simulink model "Mohinhmoix"  (R2018a)
settings: Solver=ode5  StartTime=0.0  StopTime=100  FixedStep=0.05  RelTol=1e-3
libraries: simulink x2
settings Model: PacingRate=10  Creator=Hungs  LastModifiedBy=Hungs

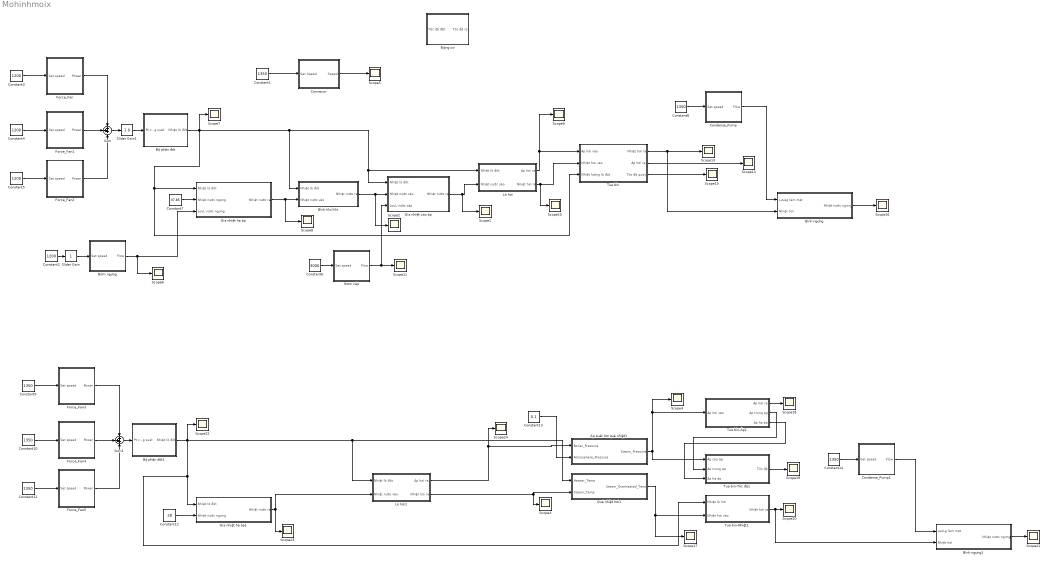
== system Mohinhmoix ==
  Bình khử khí : Subsystem
  Bình ngưng : Subsystem
  Bình ngưng1 : Subsystem
  Bơm cấp : Subsystem
      mask Display: image('C:\Program Files\MATLAB\ThermalElectricity\Maskicon\Pump.png');
  Bơm ngưng : Subsystem
      mask Display: image('C:\Program Files\MATLAB\ThermalElectricity\Maskicon\Pump.png');
  Bộ phận đốt : Subsystem
      mask Display: image('C:\Program Files\MATLAB\ThermalElectricity\Maskicon\Furnace.png');
  Bộ phận đốt1 : Subsystem
      mask Display: image('C:\Program Files\MATLAB\ThermalElectricity\Maskicon\Furnace.png');
  Condense_Pump : Subsystem
      mask Display: image('C:\Program Files\MATLAB\ThermalElectricity\Maskicon\Pump.png');
  Condense_Pump1 : Subsystem
      mask Display: image('C:\Program Files\MATLAB\ThermalElectricity\Maskicon\Pump.png');
  Constant{1,8..11,14} (6 alike) : Constant  Value=1350
  Constant12 : Constant  Value=28
  Constant13 : Constant  Value=0.1
  Constant{2..5} (4 alike) : Constant  Value=1200
  Constant6 : Constant  Value=3000
  Constant7 : Constant  Value=37.85
  Conveyor : Subsystem
      mask Display: image('C:\Program Files\MATLAB\ThermalElectricity\Maskicon\conveyor.png');
  Force_Fan : Subsystem
      mask Display: image('C:\Program Files\MATLAB\ThermalElectricity\Maskicon\Fan.png');
  Force_Fan1 : Subsystem
      mask Display: image('C:\Program Files\MATLAB\ThermalElectricity\Maskicon\Fan.png');
  Force_Fan2 : Subsystem
      mask Display: image('C:\Program Files\MATLAB\ThermalElectricity\Maskicon\Fan.png');
  Force_Fan3 : Subsystem
      mask Display: image('C:\Program Files\MATLAB\ThermalElectricity\Maskicon\Fan.png');
  Force_Fan4 : Subsystem
      mask Display: image('C:\Program Files\MATLAB\ThermalElectricity\Maskicon\Fan.png');
  Force_Fan5 : Subsystem
      mask Display: image('C:\Program Files\MATLAB\ThermalElectricity\Maskicon\Fan.png');
  Gia nhiệt cao áp : Subsystem
  Gia nhiệt hạ áp : Subsystem
  Gia nhiệt hạ áp1 : Subsystem
  Lò hơi : Subsystem
  Lò hơi1 : Subsystem
  Quá nhiệt hơi1 : Subsystem
  Scope{1..11,13..24} (23 alike) : Scope
  Slider Gain : simulink/Math Operations/Slider Gain  gain=1  low=0  high=2
  Slider Gain1 : simulink/Math Operations/Slider Gain  gain=1.0  low=0  high=2
  Sum : Sum  Inputs=+++
  Sum1 : Sum  Inputs=+++
  Tua bin : Subsystem
  Tua bin-Nhiệt1 : Subsystem
  Tua bin-Tốc độ1 : Subsystem
  Tua bin-Áp1 : Subsystem
  Áp suất hơi quá nhiệt1 : Subsystem
  Động cơ : Subsystem
  wires:
  Constant1/1 -> Conveyor/1(Set Speed)
  Conveyor/1(Speed) -> Scope5/1
  Constant2/1 -> Slider Gain/1
  Bơm ngưng/1(Flow) -> Scope6/1, Gia nhiệt hạ áp/3(LưuL nước ngưng)
  Force_Fan/1(Power) -> Sum/1
  Constant3/1 -> Force_Fan/1(Set speed)
  Constant4/1 -> Force_Fan1/1(Set speed)
  Force_Fan2/1(Power) -> Sum/3
  Constant5/1 -> Force_Fan2/1(Set speed)
  Sum/1 -> Slider Gain1/1
  Force_Fan1/1(Power) -> Sum/2
  Lò hơi/1(Áp hơi ra) -> Scope9/1, Tua bin/1(Áp hơi vào)
  Lò hơi/2(Nhiệt hơi ra) -> Scope10/1, Tua bin/2(Nhiệt hơi vào)
  Tua bin/1(Nhiệt hơi ra) -> Bình ngưng/2(Nhiệt hơi), Scope13/1
  Tua bin/2(Áp hơi ra) -> Scope14/1
  Tua bin/3(Tốc độ quay) -> Scope15/1
  Constant8/1 -> Condense_Pump/1(Set speed)
  Condense_Pump/1(Flow) -> Bình ngưng/1(LưuLg làm mát)
  Bình ngưng/1(Nhiệt nước ngưng) -> Scope16/1
  Constant12/1 -> Gia nhiệt hạ áp1/2(Nhiệt nước ngưng)
  Bình ngưng1/1(Nhiệt nước ngưng) -> Scope21/1
  Constant14/1 -> Condense_Pump1/1(Set speed)
  Tua bin-Nhiệt1/1(Nhiệt hơi ra) -> Bình ngưng1/2(Nhiệt hơi), Scope20/1
  Lò hơi1/2(Nhiệt hơi ra) -> Quá nhiệt hơi1/2(Steam_Temp), Scope3/1
  Constant10/1 -> Force_Fan4/1(Set speed)
  Tua bin-Áp1/1(Áp hơi ra) -> Scope18/1
  Constant11/1 -> Force_Fan5/1(Set speed)
  Condense_Pump1/1(Flow) -> Bình ngưng1/1(LưuLg làm mát)
  Force_Fan5/1(Power) -> Sum1/3
  Bộ phận đốt1/1(Nhiệt lò đốt) -> Quá nhiệt hơi1/1(Heater_Temp), Lò hơi1/1(Nhiệt lò đốt), Tua bin-Nhiệt1/1(Nhiệt lò hơi), Gia nhiệt hạ áp1/1(Nhiệt lò đốt), Scope22/1
  Quá nhiệt hơi1/1(Steam_Overheated_Temp) -> Tua bin-Nhiệt1/2(Nhiệt hơi vào), Scope17/1
  Constant13/1 -> Áp suất hơi quá nhiệt1/2(Atmosphere_Pressure)
  Tua bin-Áp1/3(Áp hạ áp) -> Tua bin-Tốc độ1/3(Áp hạ áp)
  Force_Fan4/1(Power) -> Sum1/2
  Áp suất hơi quá nhiệt1/1(Steam_Pressure) -> Tua bin-Tốc độ1/1(Áp cao áp), Tua bin-Áp1/1(Áp hơi vào), Scope4/1
  Gia nhiệt hạ áp1/1(Nhiệt nước ra) -> Lò hơi1/2(Nhiệt nước vào), Scope23/1
  Constant9/1 -> Force_Fan3/1(Set speed)
  Sum1/1 -> Bộ phận đốt1/1(Pt công suất)
  Force_Fan3/1(Power) -> Sum1/1
  Lò hơi1/1(Áp hơi ra) -> Áp suất hơi quá nhiệt1/1(Boiler_Pressure), Scope24/1
  Tua bin-Áp1/2(Áp trung áp) -> Tua bin-Tốc độ1/2(Áp trung áp)
  Tua bin-Tốc độ1/1(Tốc độ) -> Scope19/1
  Constant7/1 -> Gia nhiệt hạ áp/2(Nhiệt nước ngưng)
  Slider Gain/1 -> Bơm ngưng/1(Set speed)
  Slider Gain1/1 -> Bộ phận đốt/1(Pt công suất)
  Bộ phận đốt/1(Nhiệt lò đốt) -> Bình khử khí/1(Nhiệt lò đốt), Lò hơi/1(Nhiệt lò đốt), Gia nhiệt cao áp/1(Nhiệt lò đốt), Tua bin/3(Nhiệt lượng lò đốt), Gia nhiệt hạ áp/1(Nhiệt lò đốt), Scope7/1
  Gia nhiệt hạ áp/1(Nhiệt nước ra) -> Bình khử khí/2(Nhiệt nước vào), Scope8/1
  Bình khử khí/1(Nhiệt nước ra) -> Scope2/1, Gia nhiệt cao áp/2(Nhiệt nước vào)
  Constant6/1 -> Bơm cấp/1(Set speed)
  Bơm cấp/1(Flow) -> Scope11/1, Gia nhiệt cao áp/3(LưuL nước cấp)
  Gia nhiệt cao áp/1(Nhiệt nước ra) -> Scope1/1, Lò hơi/2(Nhiệt nước vào)

== system Mohinhmoix/Bình khử khí ==
  Nhiệt lò đốt : Inport
  Nhiệt nước vào : Inport  Port=2
  Gia nhiệt cao áp : TransferFcn  Numerator=[0.0435]  Denominator=[8 1]
  Sum : Sum  Inputs=|++
  Nhiệt nước ra : Outport
  wires:
  Nhiệt lò đốt/1 -> Gia nhiệt cao áp/1
  Nhiệt nước vào/1 -> Sum/1
  Gia nhiệt cao áp/1 -> Sum/2
  Sum/1 -> Nhiệt nước ra/1

== system Mohinhmoix/Bình ngưng ==
  LưuLg làm mát : Inport
  Nhiệt hơi : Inport  Port=2
  Ngưng tụ : TransferFcn  Numerator=[4.454]  Denominator=[12 1]
  Sum : Sum  Inputs=|+-
  Nhiệt nước ngưng : Outport
  wires:
  Sum/1 -> Nhiệt nước ngưng/1
  Ngưng tụ/1 -> Sum/2
  Nhiệt hơi/1 -> Sum/1
  LưuLg làm mát/1 -> Ngưng tụ/1

== system Mohinhmoix/Bình ngưng1 ==
  LưuLg làm mát : Inport
  Nhiệt hơi : Inport  Port=2
  Ngưng tụ : TransferFcn  Numerator=[5]  Denominator=[12 1]
  Sum : Sum  Inputs=|+-
  Nhiệt nước ngưng : Outport
  wires:
  Sum/1 -> Nhiệt nước ngưng/1
  Ngưng tụ/1 -> Sum/2
  Nhiệt hơi/1 -> Sum/1
  LưuLg làm mát/1 -> Ngưng tụ/1

== system Mohinhmoix/Bơm cấp ==
  Set speed : Inport
  Heat_Flow : TransferFcn  Numerator=[0.195]  Denominator=[10 1]
  Motor : TransferFcn  Denominator=[1 1 1]
  Flow : Outport
  wires:
  Motor/1 -> Heat_Flow/1
  Set speed/1 -> Motor/1
  Heat_Flow/1 -> Flow/1

== system Mohinhmoix/Bơm ngưng ==
  Set speed : Inport
  Heat_Flow : TransferFcn  Numerator=[0.512]  Denominator=[10 1]
  Motor : TransferFcn  Denominator=[1 1 1]
  Flow : Outport
  wires:
  Heat_Flow/1 -> Flow/1
  Set speed/1 -> Motor/1
  Motor/1 -> Heat_Flow/1

== system Mohinhmoix/Bộ phận đốt ==
  Pt công suất : Inport
  Vòi đốt : TransferFcn  Numerator=[1687.5]  Denominator=[5 1]
  Nhiệt lò đốt : Outport
  wires:
  Vòi đốt/1 -> Nhiệt lò đốt/1
  Pt công suất/1 -> Vòi đốt/1

== system Mohinhmoix/Bộ phận đốt1 ==
  Pt công suất : Inport
  Vòi đốt : TransferFcn  Numerator=[1350]  Denominator=[5 1]
  Nhiệt lò đốt : Outport
  wires:
  Vòi đốt/1 -> Nhiệt lò đốt/1
  Pt công suất/1 -> Vòi đốt/1

== system Mohinhmoix/Condense_Pump ==
  Set speed : Inport
  Condense_Flow : TransferFcn  Numerator=[0.012]  Denominator=[6 1]
  Motor : TransferFcn  Denominator=[1 1 1]
  Flow : Outport
  wires:
  Motor/1 -> Condense_Flow/1
  Set speed/1 -> Motor/1
  Condense_Flow/1 -> Flow/1

== system Mohinhmoix/Condense_Pump1 ==
  Set speed : Inport
  Condense_Flow : TransferFcn  Numerator=[0.012]  Denominator=[6 1]
  Motor : TransferFcn  Denominator=[1 1 1]
  Flow : Outport
  wires:
  Motor/1 -> Condense_Flow/1
  Set speed/1 -> Motor/1
  Condense_Flow/1 -> Flow/1

== system Mohinhmoix/Conveyor ==
  Set Speed : Inport
  Motor_1 : TransferFcn  Denominator=[1 1 1]
  Speed : Outport
  wires:
  Set Speed/1 -> Motor_1/1
  Motor_1/1 -> Speed/1

== system Mohinhmoix/Force_Fan ==
  Set speed : Inport
  Heat_Power : TransferFcn  Numerator=[0.000222]  Denominator=[3 1]
  Motor : TransferFcn  Denominator=[1 1 1]
  Power : Outport
  wires:
  Motor/1 -> Heat_Power/1
  Set speed/1 -> Motor/1
  Heat_Power/1 -> Power/1

== system Mohinhmoix/Force_Fan1 ==
  Set speed : Inport
  Heat_Power : TransferFcn  Numerator=[0.000222]  Denominator=[3 1]
  Motor : TransferFcn  Denominator=[1 1 1]
  Power : Outport
  wires:
  Heat_Power/1 -> Power/1
  Set speed/1 -> Motor/1
  Motor/1 -> Heat_Power/1

== system Mohinhmoix/Force_Fan2 ==
  Set speed : Inport
  Heat_Power : TransferFcn  Numerator=[0.000222]  Denominator=[3 1]
  Motor : TransferFcn  Denominator=[1 1 1]
  Power : Outport
  wires:
  Motor/1 -> Heat_Power/1
  Set speed/1 -> Motor/1
  Heat_Power/1 -> Power/1

== system Mohinhmoix/Force_Fan3 ==
  Set speed : Inport
  Heat_Power : TransferFcn  Numerator=[0.00025]  Denominator=[3 1]
  Motor : TransferFcn  Denominator=[1 1 1]
  Power : Outport
  wires:
  Motor/1 -> Heat_Power/1
  Set speed/1 -> Motor/1
  Heat_Power/1 -> Power/1

== system Mohinhmoix/Force_Fan4 ==
  Set speed : Inport
  Heat_Power : TransferFcn  Numerator=[0.00025]  Denominator=[3 1]
  Motor : TransferFcn  Denominator=[1 1 1]
  Power : Outport
  wires:
  Heat_Power/1 -> Power/1
  Set speed/1 -> Motor/1
  Motor/1 -> Heat_Power/1

== system Mohinhmoix/Force_Fan5 ==
  Set speed : Inport
  Heat_Power : TransferFcn  Numerator=[0.00025]  Denominator=[3 1]
  Motor : TransferFcn  Denominator=[1 1 1]
  Power : Outport
  wires:
  Motor/1 -> Heat_Power/1
  Set speed/1 -> Motor/1
  Heat_Power/1 -> Power/1

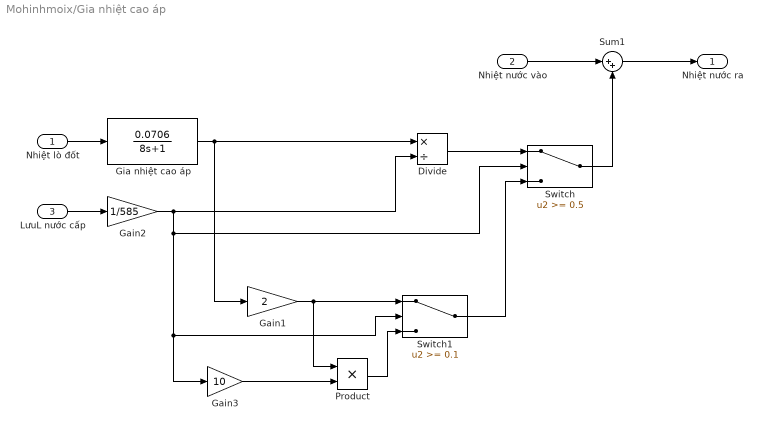
== system Mohinhmoix/Gia nhiệt cao áp ==
  Nhiệt lò đốt : Inport
  Nhiệt nước vào : Inport  Port=2
  LưuL nước cấp : Inport  Port=3
  Divide : Product  Inputs=*/
  Gain1 : Gain  Gain=2
  Gain2 : Gain  Gain=1/585
  Gain3 : Gain  Gain=10
  Gia nhiệt cao áp : TransferFcn  Numerator=[0.0706]  Denominator=[8 1]
  Product : Product
  Sum1 : Sum  Inputs=|++
  Switch : Switch  Threshold=0.5
  Switch1 : Switch  Threshold=0.1
  Nhiệt nước ra : Outport
  wires:
  Nhiệt lò đốt/1 -> Gia nhiệt cao áp/1
  Switch1/1 -> Switch/3
  Sum1/1 -> Nhiệt nước ra/1
  Switch/1 -> Sum1/2
  Nhiệt nước vào/1 -> Sum1/1
  Gain1/1 -> Switch1/1, Product/1
  Gain3/1 -> Product/2
  Product/1 -> Switch1/3
  Gia nhiệt cao áp/1 -> Divide/1, Gain1/1
  Gain2/1 -> Gain3/1, Switch1/2, Switch/2, Divide/2
  LưuL nước cấp/1 -> Gain2/1
  Divide/1 -> Switch/1

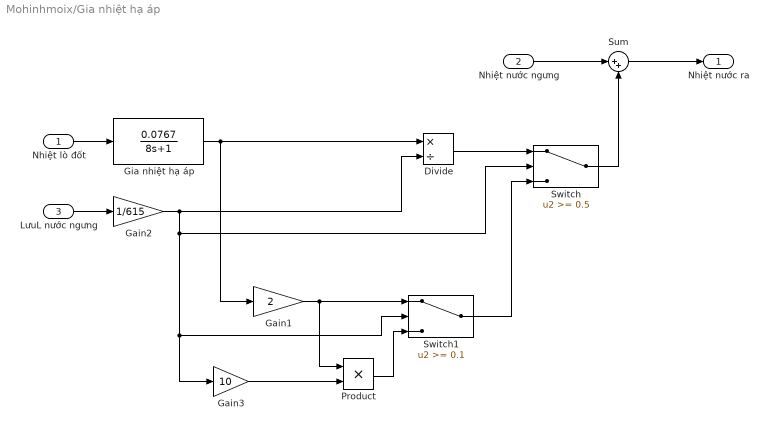
== system Mohinhmoix/Gia nhiệt hạ áp ==
  Nhiệt lò đốt : Inport
  Nhiệt nước ngưng : Inport  Port=2
  LưuL nước ngưng : Inport  Port=3
  Divide : Product  Inputs=*/
  Gain1 : Gain  Gain=2
  Gain2 : Gain  Gain=1/615
  Gain3 : Gain  Gain=10
  Gia nhiệt hạ áp : TransferFcn  Numerator=[0.0767]  Denominator=[8 1]
  Product : Product
  Sum : Sum  Inputs=|++
  Switch : Switch  Threshold=0.5
  Switch1 : Switch  Threshold=0.1
  Nhiệt nước ra : Outport
  wires:
  Sum/1 -> Nhiệt nước ra/1
  Nhiệt nước ngưng/1 -> Sum/1
  Nhiệt lò đốt/1 -> Gia nhiệt hạ áp/1
  Gia nhiệt hạ áp/1 -> Divide/1, Gain1/1
  Gain2/1 -> Gain3/1, Switch1/2, Switch/2, Divide/2
  Gain1/1 -> Switch1/1, Product/1
  Switch1/1 -> Switch/3
  Gain3/1 -> Product/2
  Product/1 -> Switch1/3
  Divide/1 -> Switch/1
  Switch/1 -> Sum/2
  LưuL nước ngưng/1 -> Gain2/1

== system Mohinhmoix/Gia nhiệt hạ áp1 ==
  Nhiệt lò đốt : Inport
  Nhiệt nước ngưng : Inport  Port=2
  Gia nhiệt hạ áp : TransferFcn  Numerator=[0.053]  Denominator=[8 1]
  Sum : Sum  Inputs=|++
  Nhiệt nước ra : Outport
  wires:
  Nhiệt lò đốt/1 -> Gia nhiệt hạ áp/1
  Nhiệt nước ngưng/1 -> Sum/1
  Gia nhiệt hạ áp/1 -> Sum/2
  Sum/1 -> Nhiệt nước ra/1

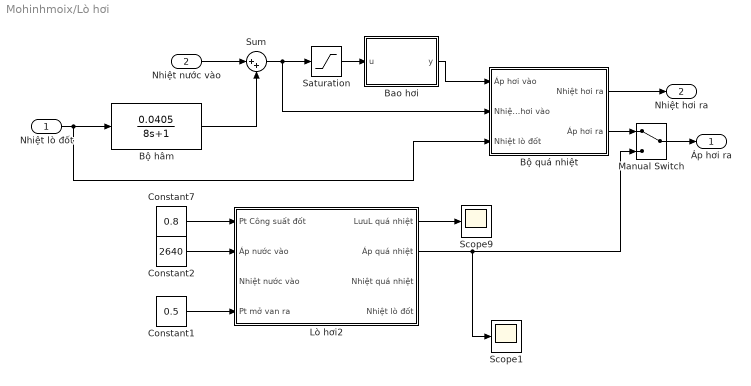
== system Mohinhmoix/Lò hơi ==
  Nhiệt lò đốt : Inport
  Nhiệt nước vào : Inport  Port=2
  Bao hơi : MATLAB Function  TreatAsAtomicUnit=on
  Bộ hâm : TransferFcn  Numerator=[0.0405]  Denominator=[8 1]
  Bộ quá nhiệt : Subsystem
  Constant1 : Constant  Value=0.5
  Constant2 : Constant  Value=2640
  Constant7 : Constant  Value=0.8
  Lò hơi2 : Subsystem
  Manual Switch : ManualSwitch
  Saturation : Saturate  UpperLimit=425  LowerLimit=0
  Scope1 : Scope
  Scope9 : Scope
  Sum : Sum  Inputs=|++
  Áp hơi ra : Outport
  Nhiệt hơi ra : Outport  Port=2
  wires:
  Sum/1 -> Bộ quá nhiệt/2(Nhiệt hơi vào), Saturation/1
  Bộ hâm/1 -> Sum/2
  Nhiệt nước vào/1 -> Sum/1
  Nhiệt lò đốt/1 -> Bộ quá nhiệt/3(Nhiệt lò đốt), Bộ hâm/1
  Bao hơi/1(y) -> Bộ quá nhiệt/1(Áp hơi vào)
  Bộ quá nhiệt/1(Nhiệt hơi ra) -> Nhiệt hơi ra/1
  Saturation/1 -> Bao hơi/1(u)
  Constant7/1 -> Lò hơi2/1(Pt Công suất đốt)
  Constant1/1 -> Lò hơi2/4(Pt mở van ra)
  Constant2/1 -> Lò hơi2/2(Áp nước vào)
  Lò hơi2/2(Áp quá nhiệt) -> Manual Switch/2, Scope1/1
  Lò hơi2/1(LưuL quá nhiệt) -> Scope9/1
  Bộ quá nhiệt/2(Áp hơi ra) -> Manual Switch/1
  Manual Switch/1 -> Áp hơi ra/1

== system Mohinhmoix/Lò hơi1 ==
  Nhiệt lò đốt : Inport
  Nhiệt nước vào : Inport  Port=2
  Bao hơi : MATLAB Function  TreatAsAtomicUnit=on
  Bộ hâm : TransferFcn  Numerator=[0.185]  Denominator=[8 1]
  Sum : Sum  Inputs=|++
  Áp hơi ra : Outport
  Nhiệt hơi ra : Outport  Port=2
  wires:
  Sum/1 -> Nhiệt hơi ra/1, Bao hơi/1(u)
  Bộ hâm/1 -> Sum/2
  Nhiệt nước vào/1 -> Sum/1
  Nhiệt lò đốt/1 -> Bộ hâm/1
  Bao hơi/1(y) -> Áp hơi ra/1

== system Mohinhmoix/Quá nhiệt hơi1 ==
  Heater_Temp : Inport
  Steam_Temp : Inport  Port=2
  Sum : Sum  Inputs=|++
  Water_Heat_Absorbing : TransferFcn  Numerator=[0.146]  Denominator=[6 1]
  Steam_Overheated_Temp : Outport
  wires:
  Sum/1 -> Steam_Overheated_Temp/1
  Water_Heat_Absorbing/1 -> Sum/2
  Steam_Temp/1 -> Sum/1
  Heater_Temp/1 -> Water_Heat_Absorbing/1

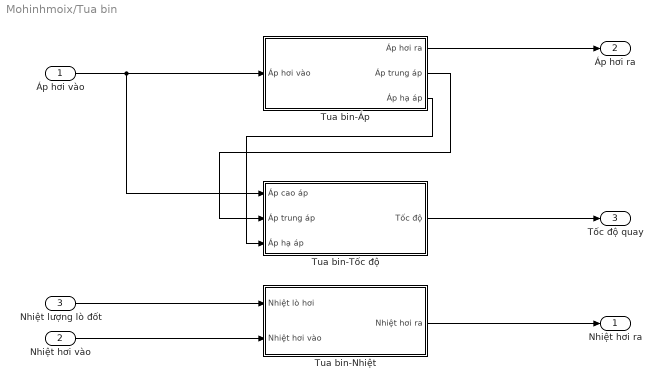
== system Mohinhmoix/Tua bin ==
  Áp hơi vào : Inport
  Nhiệt hơi vào : Inport  Port=2
  Nhiệt lượng lò đốt : Inport  Port=3
  Tua bin-Nhiệt : Subsystem
  Tua bin-Tốc độ : Subsystem
  Tua bin-Áp : Subsystem
  Nhiệt hơi ra : Outport
  Áp hơi ra : Outport  Port=2
  Tốc độ quay : Outport  Port=3
  wires:
  Tua bin-Áp/3(Áp hạ áp) -> Tua bin-Tốc độ/3(Áp hạ áp)
  Tua bin-Áp/2(Áp trung áp) -> Tua bin-Tốc độ/2(Áp trung áp)
  Áp hơi vào/1 -> Tua bin-Tốc độ/1(Áp cao áp), Tua bin-Áp/1(Áp hơi vào)
  Nhiệt hơi vào/1 -> Tua bin-Nhiệt/2(Nhiệt hơi vào)
  Tua bin-Nhiệt/1(Nhiệt hơi ra) -> Nhiệt hơi ra/1
  Tua bin-Áp/1(Áp hơi ra) -> Áp hơi ra/1
  Tua bin-Tốc độ/1(Tốc độ) -> Tốc độ quay/1
  Nhiệt lượng lò đốt/1 -> Tua bin-Nhiệt/1(Nhiệt lò hơi)

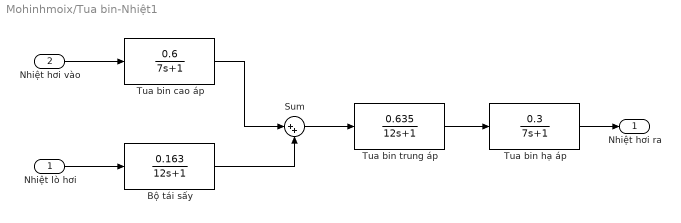
== system Mohinhmoix/Tua bin-Nhiệt1 ==
  Nhiệt lò hơi : Inport
  Nhiệt hơi vào : Inport  Port=2
  Bộ tái sấy : TransferFcn  Numerator=[0.163]  Denominator=[12 1]
  Sum : Sum  Inputs=|++
  Tua bin cao áp : TransferFcn  Numerator=[0.6]  Denominator=[7 1]
  Tua bin hạ áp : TransferFcn  Numerator=[0.3]  Denominator=[7 1]
  Tua bin trung áp : TransferFcn  Numerator=[0.635]  Denominator=[12 1]
  Nhiệt hơi ra : Outport
  wires:
  Nhiệt lò hơi/1 -> Bộ tái sấy/1
  Bộ tái sấy/1 -> Sum/2
  Nhiệt hơi vào/1 -> Tua bin cao áp/1
  Tua bin cao áp/1 -> Sum/1
  Sum/1 -> Tua bin trung áp/1
  Tua bin trung áp/1 -> Tua bin hạ áp/1
  Tua bin hạ áp/1 -> Nhiệt hơi ra/1

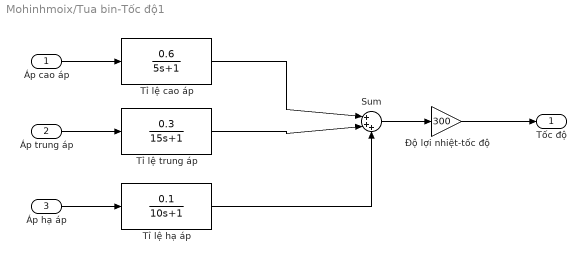
== system Mohinhmoix/Tua bin-Tốc độ1 ==
  Áp cao áp : Inport
  Áp trung áp : Inport  Port=2
  Áp hạ áp : Inport  Port=3
  Sum : Sum  Inputs=|+++
  Tỉ lệ cao áp : TransferFcn  Numerator=[0.6]  Denominator=[5 1]
  Tỉ lệ hạ áp : TransferFcn  Numerator=[0.1]  Denominator=[10 1]
  Tỉ lệ trung áp : TransferFcn  Numerator=[0.3]  Denominator=[15 1]
  Độ lợi nhiệt-tốc độ : Gain  Gain=300
  Tốc độ : Outport
  wires:
  Áp cao áp/1 -> Tỉ lệ cao áp/1
  Tỉ lệ cao áp/1 -> Sum/1
  Sum/1 -> Độ lợi nhiệt-tốc độ/1
  Áp trung áp/1 -> Tỉ lệ trung áp/1
  Áp hạ áp/1 -> Tỉ lệ hạ áp/1
  Tỉ lệ trung áp/1 -> Sum/2
  Tỉ lệ hạ áp/1 -> Sum/3
  Độ lợi nhiệt-tốc độ/1 -> Tốc độ/1

== system Mohinhmoix/Tua bin-Áp1 ==
  Áp hơi vào : Inport
  Tua bin cao áp : TransferFcn  Numerator=[0.23]  Denominator=[1 1]
  Tua bin hạ áp : TransferFcn  Numerator=[0.011]  Denominator=[2 1]
  Tua bin trung áp : TransferFcn  Numerator=[0.23]  Denominator=[4 1]
  Áp hơi ra : Outport
  Áp trung áp : Outport  Port=2
  Áp hạ áp : Outport  Port=3
  wires:
  Tua bin hạ áp/1 -> Áp hơi ra/1
  Tua bin trung áp/1 -> Áp hạ áp/1, Tua bin hạ áp/1
  Tua bin cao áp/1 -> Áp trung áp/1, Tua bin trung áp/1
  Áp hơi vào/1 -> Tua bin cao áp/1

== system Mohinhmoix/Áp suất hơi quá nhiệt1 ==
  Boiler_Pressure : Inport
  Atmosphere_Pressure : Inport  Port=2
  Overheated_Pressure : TransferFcn  Numerator=[1.1]  Denominator=[2 1]
  Sum : Sum  Inputs=++|
  Steam_Pressure : Outport
  wires:
  Overheated_Pressure/1 -> Steam_Pressure/1
  Boiler_Pressure/1 -> Sum/2
  Sum/1 -> Overheated_Pressure/1
  Atmosphere_Pressure/1 -> Sum/1

== system Mohinhmoix/Động cơ ==
  Tốc độ đặt : Inport
  Bão hòa 2 cực : Saturate  UpperLimit=1500  LowerLimit=0
  Động cơ AC : TransferFcn  Denominator=[1 1 1]
  Tốc độ ra : Outport
  wires:
  Bão hòa 2 cực/1 -> Tốc độ ra/1
  Tốc độ đặt/1 -> Động cơ AC/1
  Động cơ AC/1 -> Bão hòa 2 cực/1

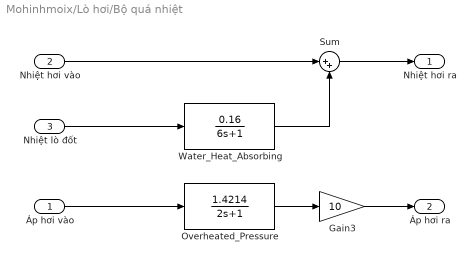
== system Mohinhmoix/Lò hơi/Bộ quá nhiệt ==
  Áp hơi vào : Inport
  Nhiệt hơi vào : Inport  Port=2
  Nhiệt lò đốt : Inport  Port=3
  Gain3 : Gain  Gain=10
  Overheated_Pressure : TransferFcn  Numerator=[1.4214]  Denominator=[2 1]
  Sum : Sum  Inputs=|++
  Water_Heat_Absorbing : TransferFcn  Numerator=[0.16]  Denominator=[6 1]
  Nhiệt hơi ra : Outport
  Áp hơi ra : Outport  Port=2
  wires:
  Sum/1 -> Nhiệt hơi ra/1
  Water_Heat_Absorbing/1 -> Sum/2
  Nhiệt hơi vào/1 -> Sum/1
  Nhiệt lò đốt/1 -> Water_Heat_Absorbing/1
  Áp hơi vào/1 -> Overheated_Pressure/1
  Overheated_Pressure/1 -> Gain3/1
  Gain3/1 -> Áp hơi ra/1

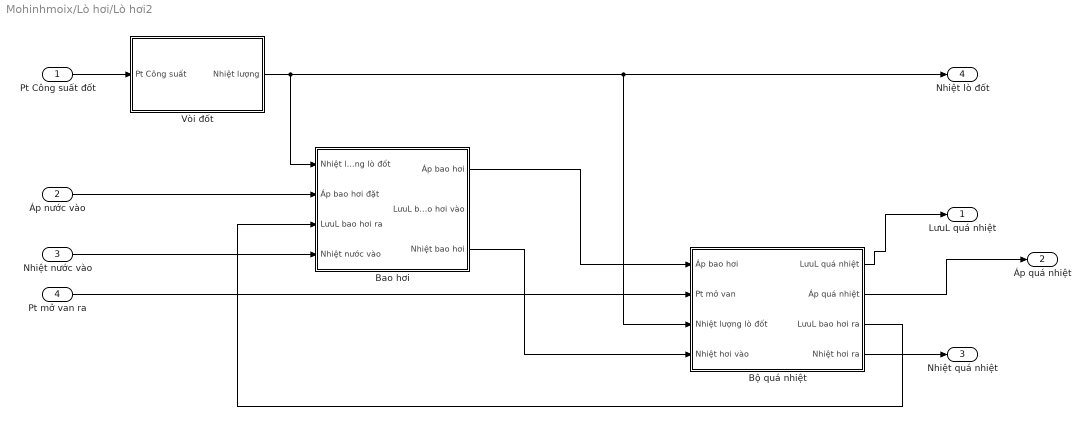
== system Mohinhmoix/Lò hơi/Lò hơi2 ==
  Pt Công suất đốt : Inport
  Áp nước vào : Inport  Port=2
  Nhiệt nước vào : Inport  Port=3
  Pt mở van ra : Inport  Port=4
  Bao hơi : Subsystem  mask{Cm=0.3, Kw=0.04, Kt=0.000025, Kh=-300, Cd=150}
      mask prompts: Cm "Hệ số hấp thụ nhiệt ống sinh hơi"; Kw "Hệ số truyền nhiệt ống sinh hơi"; Kt "Tỉ lệ áp suất - nhiệt độ trong ống sinh hơi"; Kh "Hệ số biến thiên entanpi theo áp suất bao hơi"; Cd "Thời hằng bao hơi"
  Bộ quá nhiệt : Subsystem  mask{K=44, Cs=20}
      mask prompts: K "Hệ số tụt áp"; Cs "Thời hằng bộ quá nhiệt"
  Vòi đốt : Subsystem  mask{Tf=100, Td=20}
      mask prompts: Tf "Thời hằng vòi đốt"; Td "Thời gian trễ vòi đốt"
  LưuL quá nhiệt : Outport
  Áp quá nhiệt : Outport  Port=2
  Nhiệt quá nhiệt : Outport  Port=3
  Nhiệt lò đốt : Outport  Port=4
  wires:
  Bộ quá nhiệt/1(LưuL quá nhiệt) -> LưuL quá nhiệt/1
  Bao hơi/1(Áp bao hơi) -> Bộ quá nhiệt/1(Áp bao hơi)
  Bộ quá nhiệt/3(LưuL bao hơi ra) -> Bao hơi/3(LưuL bao hơi ra)
  Pt mở van ra/1 -> Bộ quá nhiệt/2(Pt mở van)
  Áp nước vào/1 -> Bao hơi/2(Áp bao hơi đặt)
  Bộ quá nhiệt/2(Áp quá nhiệt) -> Áp quá nhiệt/1
  Nhiệt nước vào/1 -> Bao hơi/4(Nhiệt nước vào)
  Bao hơi/3(Nhiệt bao hơi) -> Bộ quá nhiệt/4(Nhiệt hơi vào)
  Bộ quá nhiệt/4(Nhiệt hơi ra) -> Nhiệt quá nhiệt/1
  Pt Công suất đốt/1 -> Vòi đốt/1(Pt Công suất)
  Vòi đốt/1(Nhiệt lượng) -> Nhiệt lò đốt/1, Bộ quá nhiệt/3(Nhiệt lượng lò đốt), Bao hơi/1(Nhiệt lượng lò đốt)

== system Mohinhmoix/Tua bin/Tua bin-Nhiệt ==
  Nhiệt lò hơi : Inport
  Nhiệt hơi vào : Inport  Port=2
  Bộ tái sấy : TransferFcn  Numerator=[0.195]  Denominator=[12 1]
  Sum : Sum  Inputs=|++
  Tua bin cao áp : TransferFcn  Numerator=[0.582]  Denominator=[7 1]
  Tua bin hạ áp : TransferFcn  Numerator=[0.3]  Denominator=[7 1]
  Tua bin trung áp : TransferFcn  Numerator=[0.574]  Denominator=[12 1]
  Nhiệt hơi ra : Outport
  wires:
  Tua bin hạ áp/1 -> Nhiệt hơi ra/1
  Tua bin trung áp/1 -> Tua bin hạ áp/1
  Sum/1 -> Tua bin trung áp/1
  Tua bin cao áp/1 -> Sum/1
  Nhiệt hơi vào/1 -> Tua bin cao áp/1
  Bộ tái sấy/1 -> Sum/2
  Nhiệt lò hơi/1 -> Bộ tái sấy/1

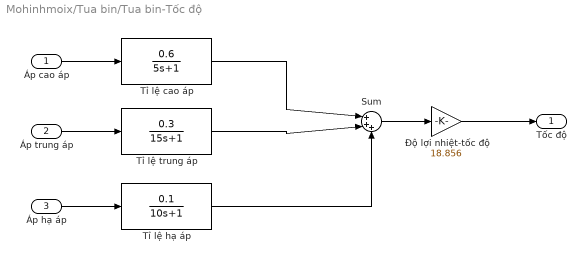
== system Mohinhmoix/Tua bin/Tua bin-Tốc độ ==
  Áp cao áp : Inport
  Áp trung áp : Inport  Port=2
  Áp hạ áp : Inport  Port=3
  Sum : Sum  Inputs=|+++
  Tỉ lệ cao áp : TransferFcn  Numerator=[0.6]  Denominator=[5 1]
  Tỉ lệ hạ áp : TransferFcn  Numerator=[0.1]  Denominator=[10 1]
  Tỉ lệ trung áp : TransferFcn  Numerator=[0.3]  Denominator=[15 1]
  Độ lợi nhiệt-tốc độ : Gain  Gain=18.856
  Tốc độ : Outport
  wires:
  Áp cao áp/1 -> Tỉ lệ cao áp/1
  Tỉ lệ cao áp/1 -> Sum/1
  Sum/1 -> Độ lợi nhiệt-tốc độ/1
  Áp trung áp/1 -> Tỉ lệ trung áp/1
  Áp hạ áp/1 -> Tỉ lệ hạ áp/1
  Tỉ lệ trung áp/1 -> Sum/2
  Tỉ lệ hạ áp/1 -> Sum/3
  Độ lợi nhiệt-tốc độ/1 -> Tốc độ/1

== system Mohinhmoix/Tua bin/Tua bin-Áp ==
  Áp hơi vào : Inport
  Tua bin cao áp : TransferFcn  Numerator=[0.18]  Denominator=[1 1]
  Tua bin hạ áp : TransferFcn  Numerator=[0.00757]  Denominator=[2 1]
  Tua bin trung áp : TransferFcn  Numerator=[0.2]  Denominator=[4 1]
  Áp hơi ra : Outport
  Áp trung áp : Outport  Port=2
  Áp hạ áp : Outport  Port=3
  wires:
  Tua bin hạ áp/1 -> Áp hơi ra/1
  Tua bin trung áp/1 -> Áp hạ áp/1, Tua bin hạ áp/1
  Tua bin cao áp/1 -> Áp trung áp/1, Tua bin trung áp/1
  Áp hơi vào/1 -> Tua bin cao áp/1

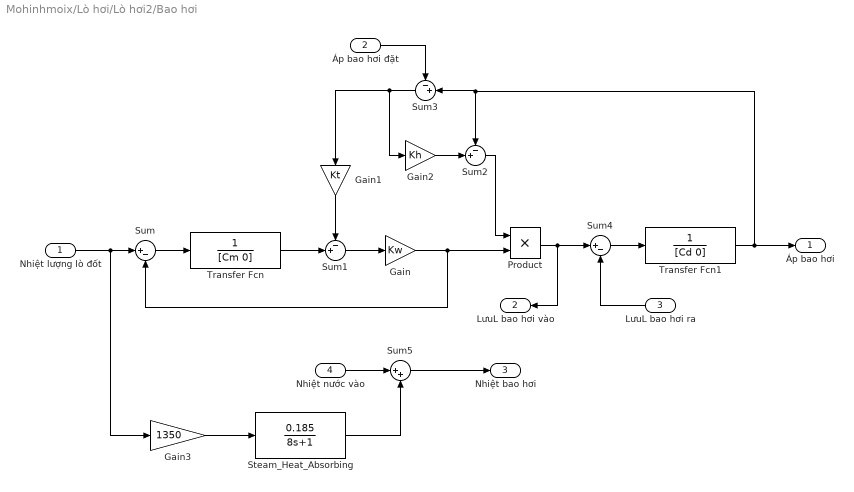
== system Mohinhmoix/Lò hơi/Lò hơi2/Bao hơi ==
  Nhiệt lượng lò đốt : Inport
  Áp bao hơi đặt : Inport  Port=2
  LưuL bao hơi ra : Inport  Port=3
  Nhiệt nước vào : Inport  Port=4
  Gain : Gain  Gain=Kw
  Gain1 : Gain  Gain=Kt
  Gain2 : Gain  Gain=Kh
  Gain3 : Gain  Gain=1350
  Product : Product
  Steam_Heat_Absorbing : TransferFcn  Numerator=[0.185]  Denominator=[8 1]
  Sum : Sum  Inputs=|+-
  Sum1 : Sum  Inputs=-+|
  Sum2 : Sum  Inputs=-+|
  Sum3 : Sum  Inputs=-+|
  Sum4 : Sum  Inputs=|+-
  Sum5 : Sum  Inputs=|++
  Transfer Fcn : TransferFcn  Denominator=[Cm 0]
  Transfer Fcn1 : TransferFcn  Denominator=[Cd 0]
  Áp bao hơi : Outport
  LưuL bao hơi vào : Outport  Port=2
  Nhiệt bao hơi : Outport  Port=3
  wires:
  Transfer Fcn/1 -> Sum1/2
  Sum1/1 -> Gain/1
  Gain/1 -> Product/2, Sum/2
  Sum/1 -> Transfer Fcn/1
  Gain1/1 -> Sum1/1
  Transfer Fcn1/1 -> Áp bao hơi/1, Sum2/1, Sum3/2
  Sum2/1 -> Product/1
  Gain2/1 -> Sum2/2
  Sum3/1 -> Gain1/1, Gain2/1
  Áp bao hơi đặt/1 -> Sum3/1
  Product/1 -> Sum4/1, LưuL bao hơi vào/1
  LưuL bao hơi ra/1 -> Sum4/2
  Sum4/1 -> Transfer Fcn1/1
  Nhiệt lượng lò đốt/1 -> Sum/1, Gain3/1
  Steam_Heat_Absorbing/1 -> Sum5/2
  Nhiệt nước vào/1 -> Sum5/1
  Sum5/1 -> Nhiệt bao hơi/1
  Gain3/1 -> Steam_Heat_Absorbing/1

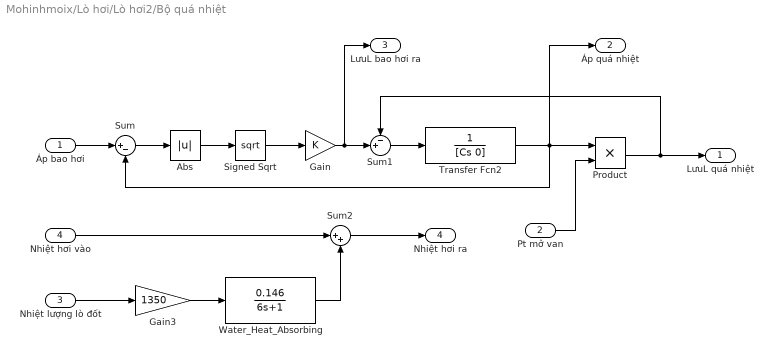
== system Mohinhmoix/Lò hơi/Lò hơi2/Bộ quá nhiệt ==
  Áp bao hơi : Inport
  Pt mở van : Inport  Port=2
  Nhiệt lượng lò đốt : Inport  Port=3
  Nhiệt hơi vào : Inport  Port=4
  Abs : Abs
  Gain : Gain  Gain=K
  Gain3 : Gain  Gain=1350
  Product : Product
  Signed Sqrt : Sqrt  SaturateOnIntegerOverflow=on
  Sum : Sum  Inputs=|+-
  Sum1 : Sum  Inputs=-+|
  Sum2 : Sum  Inputs=|++
  Transfer Fcn2 : TransferFcn  Denominator=[Cs 0]
  Water_Heat_Absorbing : TransferFcn  Numerator=[0.146]  Denominator=[6 1]
  LưuL quá nhiệt : Outport
  Áp quá nhiệt : Outport  Port=2
  LưuL bao hơi ra : Outport  Port=3
  Nhiệt hơi ra : Outport  Port=4
  wires:
  Transfer Fcn2/1 -> Áp quá nhiệt/1, Sum/2, Product/1
  Áp bao hơi/1 -> Sum/1
  Sum/1 -> Abs/1
  Abs/1 -> Signed Sqrt/1
  Signed Sqrt/1 -> Gain/1
  Pt mở van/1 -> Product/2
  Gain/1 -> LưuL bao hơi ra/1, Sum1/2
  Sum1/1 -> Transfer Fcn2/1
  Product/1 -> LưuL quá nhiệt/1, Sum1/1
  Nhiệt hơi vào/1 -> Sum2/1
  Water_Heat_Absorbing/1 -> Sum2/2
  Nhiệt lượng lò đốt/1 -> Gain3/1
  Sum2/1 -> Nhiệt hơi ra/1
  Gain3/1 -> Water_Heat_Absorbing/1

== system Mohinhmoix/Lò hơi/Lò hơi2/Vòi đốt ==
  Pt Công suất : Inport
  Furnace : TransferFcn  Denominator=[Tf 1]
  Transport Delay : TransportDelay  DelayTime=Td
  Nhiệt lượng : Outport
  wires:
  Pt Công suất/1 -> Furnace/1
  Furnace/1 -> Transport Delay/1
  Transport Delay/1 -> Nhiệt lượng/1

== matlab function Mohinhmoix/Lò hơi1/Bao hơi ==
  data: u input; y output
function y = fcn(u)
to = [17 22 27 29.95 32.89 41.53 45.82 52.57 60.08 69.12 75.87 81.33 93.5 99.62 109.32 ...
    120.24 133.56 143.64 151.87 158.86 164.98 170.44 175.39 179.92 195.08 212.42 ...
    233.89 250.39 263.98 285.86 311.03 342.34 357.04 365.80 373.70];
p = [0.00192 0.00262 0.00354 0.004 0.005 0.008 0.01 0.018 0.02 0.03 0.04 0.05 0.08 0.1 0.14 0.2 0.3 0.4 ...
    0.5 0.6 0.7 0.8 0.9 1 1.4 2 3 4 5 7 10 15 18 20 22];
y = interp1(to,p,u);

== matlab function Mohinhmoix/Lò hơi/Bao hơi ==
  data: u input; y output
function y = fcn(u)
to = [17 22 27 29.95 32.89 41.53 45.82 52.57 60.08 69.12 75.87 81.33 93.5 99.62 109.32 ...
    120.24 133.56 143.64 151.87 158.86 164.98 170.44 175.39 179.92 195.08 212.42 ...
    233.89 250.39 263.98 285.86 311.03 342.34 357.04 365.80 373.70 425];
p = [0.00192 0.00262 0.00354 0.004 0.005 0.008 0.01 0.018 0.02 0.03 0.04 0.05 0.08 0.1 0.14 0.2 0.3 0.4 ...
    0.5 0.6 0.7 0.8 0.9 1 1.4 2 3 4 5 7 10 15 18 20 22 35];
y = interp1(to,p,u);
